simulink model "test_swift_sti"  (Simulink 4.1.1)
settings: Solver=ode45  SolverMode=SingleTasking  StartTime=0.0  StopTime=0.4  FixedStep=0.02  MaxStep=0.0005  RelTol=1e-4  AbsTol=1e-4
libraries: simulink3 x3, dtlib x2
settings Model: LastModifiedBy=besselink  InitialStep=0.0005  LimitDataPoints=off  ExtModeTrigMode=oneshot  ExtModeArmWhenConnect=off

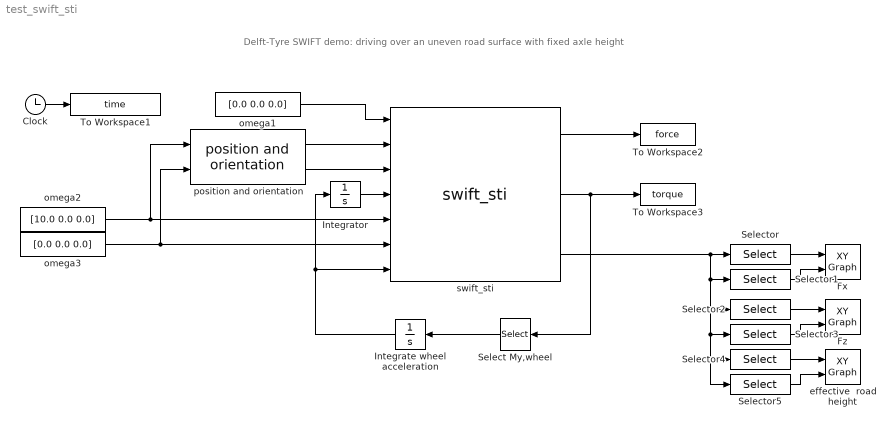
== system test_swift_sti ==
  note: Delft-Tyre SWIFT demo: driving over an uneven road surface with fixed axle height
  Clock : Clock
      settings: DisplayTime=off  Decimation=10
  Fx : simulink3/Sinks/XY Graph  xmin=0  xmax=4  ymin=-4000  ymax=4000  st=-1
  Fz : simulink3/Sinks/XY Graph  xmin=0  xmax=4  ymin=0  ymax=10000  st=-1
  Integrate wheel acceleration : Integrator  Orientation=left  ExternalReset=none  InitialConditionSource=internal  InitialCondition=10/0.3057  LimitOutput=off  UpperSaturationLimit=inf  LowerSaturationLimit=-inf  ShowSaturationPort=off  ShowStatePort=off  AbsoluteTolerance=auto
  Integrator : Integrator  ExternalReset=none  InitialConditionSource=internal  InitialCondition=0  LimitOutput=off  UpperSaturationLimit=inf  LowerSaturationLimit=-inf  ShowSaturationPort=off  ShowStatePort=off  AbsoluteTolerance=auto
  Select My,wheel : Selector  Orientation=left  InputType=Vector  ElementSrc=Internal  Elements=2  RowSrc=Internal  Rows=1  ColumnSrc=Internal  Columns=1  InputPortWidth=3
  Selector : Selector  InputType=Vector  ElementSrc=Internal  Elements=36  RowSrc=Internal  Rows=1  ColumnSrc=Internal  Columns=1  InputPortWidth=40
  Selector1 : Selector  InputType=Vector  ElementSrc=Internal  Elements=4  RowSrc=Internal  Rows=1  ColumnSrc=Internal  Columns=1  InputPortWidth=40
  Selector2 : Selector  InputType=Vector  ElementSrc=Internal  Elements=36  RowSrc=Internal  Rows=1  ColumnSrc=Internal  Columns=1  InputPortWidth=40
  Selector3 : Selector  InputType=Vector  ElementSrc=Internal  Elements=6  RowSrc=Internal  Rows=1  ColumnSrc=Internal  Columns=1  InputPortWidth=40
  Selector4 : Selector  InputType=Vector  ElementSrc=Internal  Elements=36  RowSrc=Internal  Rows=1  ColumnSrc=Internal  Columns=1  InputPortWidth=40
  Selector5 : Selector  InputType=Vector  ElementSrc=Internal  Elements=37  RowSrc=Internal  Rows=1  ColumnSrc=Internal  Columns=1  InputPortWidth=40
  To Workspace1 : ToWorkspace  VariableName=time  SampleTime=-1  SaveFormat=Array
  To Workspace2 : ToWorkspace  VariableName=force  SampleTime=-1  SaveFormat=Array
  To Workspace3 : ToWorkspace  VariableName=torque  SampleTime=-1  SaveFormat=Array
  effective  road height : simulink3/Sinks/XY Graph  xmin=0  xmax=4  ymin=-0.05  ymax=0.05  st=-1
  omega1 : Constant  Value=[0.0 0.0 0.0]
  omega2 : Constant  Value=[10.0 0.0 0.0]
  omega3 : Constant  Value=[0.0 0.0 0.0]
  position and orientation : dtlib/position and orientation  init_pos=[0 0 0.29]  init_angle=[0 0 0]
  swift_sti : dtlib/swift_sti  idtyre=1  use_mode=124  tpfname='swt_car205_60R15.tir'  road_popup=Data file (effective inputs)  rdfname='swt_road.rdf'
  wires:
  omega1/1 -> swift_sti/1
  Integrator/1 -> swift_sti/4
  swift_sti/1 -> To Workspace2/1
  swift_sti/2 -> Select My,wheel/1, To Workspace3/1
  Clock/1 -> To Workspace1/1
  Integrate wheel acceleration/1 -> swift_sti/7, Integrator/1
  Select My,wheel/1 -> Integrate wheel acceleration/1
  position and orientation/1 -> swift_sti/2
  position and orientation/2 -> swift_sti/3
  omega2/1 -> swift_sti/5, position and orientation/1
  omega3/1 -> swift_sti/6, position and orientation/2
  swift_sti/3 -> Selector/1, Selector1/1, Selector2/1, Selector3/1, Selector5/1, Selector4/1
  Selector/1 -> Fx/1
  Selector1/1 -> Fx/2
  Selector2/1 -> Fz/1
  Selector3/1 -> Fz/2
  Selector4/1 -> effective  road height/1
  Selector5/1 -> effective  road height/2
